simulink model "Lab_2v0"  (R2022a)
settings: Solver=VariableStepAuto  StartTime=0.0  StopTime=3600  RelTol=1e-12
settings Model: Creator=yjyoo  LastModifiedBy=ACL2022_14

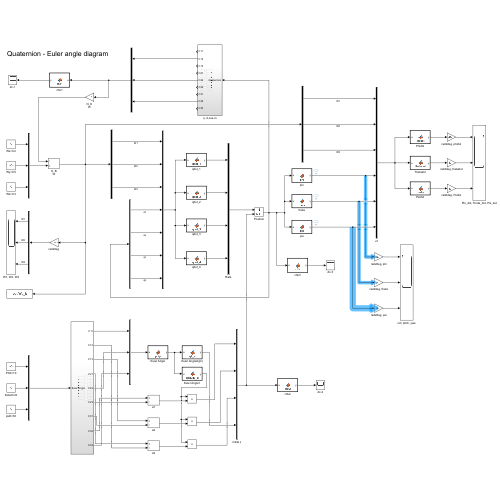
[thumbnail: Simulink's stored preview of the top-level diagram]
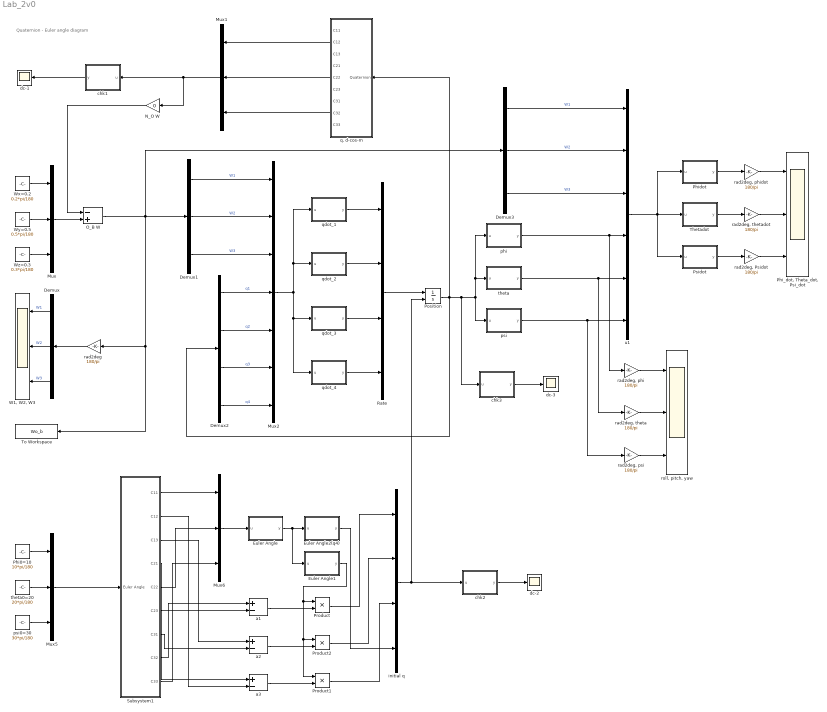
== system Lab_2v0 ==
  note: Quaternion - Euler angle diagram
  Demux : Demux  Outputs=3
  Demux1 : Demux  Outputs=3
  Demux2 : Demux
  Demux3 : Demux  Outputs=3
  Euler Angle : MATLAB Function  TreatAsAtomicUnit=on
  Euler Angle1 : MATLAB Function  TreatAsAtomicUnit=on
  Euler Angle2(q4) : MATLAB Function  TreatAsAtomicUnit=on
  Mux{,1,5..6} (4 alike) : Mux  Inputs=3
  Mux2 : Mux  Inputs=7
  N_O W : Gain  Gain=0
  O_B W : Sum  Inputs=-+
  Phi0=10 : Constant  Value=10*pi/180
  "Phi_dot, Theta_dot, Psi_dot" : Scope  NumInputPorts=3
  Phidot : MATLAB Function  TreatAsAtomicUnit=on
  Position : Integrator  InitialConditionSource=external
  Product : Product
  Product1 : Product
  Product2 : Product
  Psidot : MATLAB Function  TreatAsAtomicUnit=on
  Rate : Mux
  Subsystem1 : Subsystem
  Thetadot : MATLAB Function  TreatAsAtomicUnit=on
  To Workspace : ToWorkspace  VariableName=Wo_b  SaveFormat=Timeseries  SampleTime=-1
  "W1, W2, W3" : Scope  NumInputPorts=3
  Wx=0.2 : Constant  Value=0.2*pi/180
  Wy=0.5 : Constant  Value=0.5*pi/180
  Wz=0.3 : Constant  Value=0.3*pi/180
  a1 : Sum  Inputs=+-
  a2 : Sum  Inputs=+-
  a3 : Sum  Inputs=+-
  chk1 : MATLAB Function  TreatAsAtomicUnit=on
  chk2 : MATLAB Function  TreatAsAtomicUnit=on
  chk3 : MATLAB Function  TreatAsAtomicUnit=on
  dc-1 : Scope
  dc-2 : Scope
  dc-3 : Scope
  initial q : Mux
  phi : MATLAB Function  TreatAsAtomicUnit=on
  psi : MATLAB Function  TreatAsAtomicUnit=on
  psi0=30 : Constant  Value=30*pi/180
  q. d-cos-m : Subsystem
  qdot_1 : MATLAB Function  TreatAsAtomicUnit=on
  qdot_2 : MATLAB Function  TreatAsAtomicUnit=on
  qdot_3 : MATLAB Function  TreatAsAtomicUnit=on
  qdot_4 : MATLAB Function  TreatAsAtomicUnit=on
  rad2deg : Gain  Gain=180/pi
  "rad2deg, Psidot" : Gain  Gain=180/pi
  "rad2deg, phi" : Gain  Gain=180/pi
  "rad2deg, phidot" : Gain  Gain=180/pi
  "rad2deg, psi" : Gain  Gain=180/pi
  "rad2deg, theta" : Gain  Gain=180/pi
  "rad2deg, thetadot" : Gain  Gain=180/pi
  "roll, pitch, yaw" : Scope  NumInputPorts=3
  theta : MATLAB Function  TreatAsAtomicUnit=on
  theta0=20 : Constant  Value=20*pi/180
  u1 : Mux  Inputs=6
  wires:
  Wx=0.2/1 -> Mux/1
  Wy=0.5/1 -> Mux/2
  Wz=0.3/1 -> Mux/3
  Mux/1 -> O_B W/2
  N_O W/1 -> O_B W/1
  Mux1/1 -> N_O W/1, chk1/1(u)
  chk1/1(y) -> dc-1/1
  Demux/1 -> "W1, W2, W3"/1  "W1"
  Demux/2 -> "W1, W2, W3"/2  "W2"
  Demux/3 -> "W1, W2, W3"/3  "W3"
  O_B W/1 -> Demux1/1, Demux3/1, To Workspace/1, rad2deg/1
  Demux2/1 -> Mux2/4  "q1"
  Demux2/2 -> Mux2/5  "q2"
  Demux2/3 -> Mux2/6  "q3"
  Demux2/4 -> Mux2/7  "q4"
  Demux1/1 -> Mux2/1  "W1"
  Demux1/2 -> Mux2/2  "W2"
  Demux1/3 -> Mux2/3  "W3"
  rad2deg/1 -> Demux/1
  qdot_2/1(y) -> Rate/2
  qdot_1/1(y) -> Rate/1
  qdot_3/1(y) -> Rate/3
  qdot_4/1(y) -> Rate/4
  phi/1(y) -> "rad2deg, phi"/1, u1/4
  psi/1(y) -> "rad2deg, psi"/1, u1/6
  Demux3/1 -> u1/1  "W1"
  Demux3/2 -> u1/2  "W2"
  Demux3/3 -> u1/3  "W3"
  u1/1 -> Phidot/1(u), Psidot/1(u), Thetadot/1(u)
  "rad2deg, phidot"/1 -> "Phi_dot, Theta_dot, Psi_dot"/1
  "rad2deg, thetadot"/1 -> "Phi_dot, Theta_dot, Psi_dot"/2
  "rad2deg, Psidot"/1 -> "Phi_dot, Theta_dot, Psi_dot"/3
  Phidot/1(y) -> "rad2deg, phidot"/1
  Thetadot/1(y) -> "rad2deg, thetadot"/1
  Psidot/1(y) -> "rad2deg, Psidot"/1
  "rad2deg, psi"/1 -> "roll, pitch, yaw"/3
  "rad2deg, theta"/1 -> "roll, pitch, yaw"/2
  "rad2deg, phi"/1 -> "roll, pitch, yaw"/1
  theta/1(y) -> "rad2deg, theta"/1, u1/5
  Rate/1 -> Position/1
  Mux2/1 -> qdot_4/1(u), qdot_3/1(u), qdot_1/1(u), qdot_2/1(u)
  Position/1 -> Demux2/1, psi/1(u), phi/1(u), theta/1(u), chk3/1(u), q. d-cos-m/1(Quaternion)
  chk3/1(y) -> dc-3/1
  q. d-cos-m/2(C12) -> Mux1/1
  q. d-cos-m/5(C22) -> Mux1/2
  q. d-cos-m/8(C32) -> Mux1/3
  psi0=30/1 -> Mux5/3
  theta0=20/1 -> Mux5/2
  Phi0=10/1 -> Mux5/1
  Mux5/1 -> Subsystem1/1(Euler Angle)
  Mux6/1 -> Euler Angle/1(u)
  initial q/1 -> Position/2, chk2/1(u)
  chk2/1(y) -> dc-2/1
  Euler Angle2(q4)/1(y) -> initial q/4
  Euler Angle1/1(y) -> Product2/1, Product1/1, Product/1
  a1/1 -> Product/2
  a2/1 -> Product2/2
  a3/1 -> Product1/2
  Product/1 -> initial q/1
  Product2/1 -> initial q/2
  Product1/1 -> initial q/3
  Euler Angle/1(y) -> Euler Angle1/1(u), Euler Angle2(q4)/1(u)
  Subsystem1/8(C32) -> a1/1
  Subsystem1/6(C23) -> a1/2
  Subsystem1/3(C13) -> a2/1
  Subsystem1/7(C31) -> a2/2
  Subsystem1/4(C21) -> a3/1
  Subsystem1/2(C12) -> a3/2
  Subsystem1/1(C11) -> Mux6/1
  Subsystem1/5(C22) -> Mux6/2
  Subsystem1/9(C33) -> Mux6/3

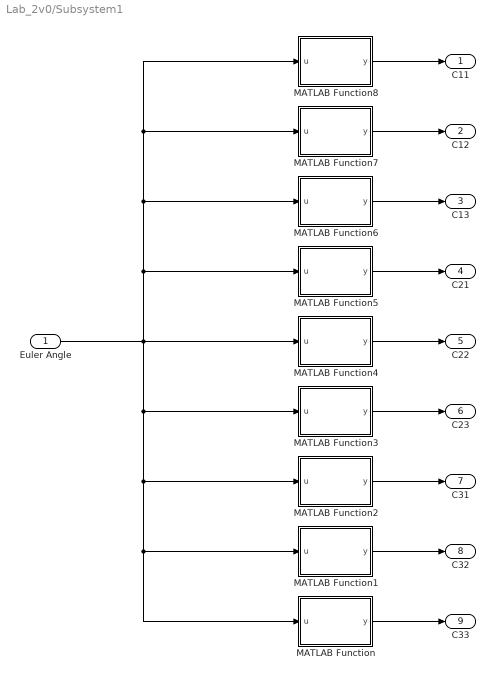
== system Lab_2v0/Subsystem1 ==
  Euler Angle : Inport
  MATLAB Function : MATLAB Function  TreatAsAtomicUnit=on
  MATLAB Function1 : MATLAB Function  TreatAsAtomicUnit=on
  MATLAB Function2 : MATLAB Function  TreatAsAtomicUnit=on
  MATLAB Function3 : MATLAB Function  TreatAsAtomicUnit=on
  MATLAB Function4 : MATLAB Function  TreatAsAtomicUnit=on
  MATLAB Function5 : MATLAB Function  TreatAsAtomicUnit=on
  MATLAB Function6 : MATLAB Function  TreatAsAtomicUnit=on
  MATLAB Function7 : MATLAB Function  TreatAsAtomicUnit=on
  MATLAB Function8 : MATLAB Function  TreatAsAtomicUnit=on
  C11 : Outport
  C12 : Outport  Port=2
  C13 : Outport  Port=3
  C21 : Outport  Port=4
  C22 : Outport  Port=5
  C23 : Outport  Port=6
  C31 : Outport  Port=7
  C32 : Outport  Port=8
  C33 : Outport  Port=9
  wires:
  Euler Angle/1 -> MATLAB Function/1(u), MATLAB Function1/1(u), MATLAB Function2/1(u), MATLAB Function3/1(u), MATLAB Function8/1(u), MATLAB Function7/1(u), MATLAB Function6/1(u), MATLAB Function5/1(u), MATLAB Function4/1(u)
  MATLAB Function/1(y) -> C33/1
  MATLAB Function1/1(y) -> C32/1
  MATLAB Function2/1(y) -> C31/1
  MATLAB Function3/1(y) -> C23/1
  MATLAB Function4/1(y) -> C22/1
  MATLAB Function5/1(y) -> C21/1
  MATLAB Function6/1(y) -> C13/1
  MATLAB Function7/1(y) -> C12/1
  MATLAB Function8/1(y) -> C11/1

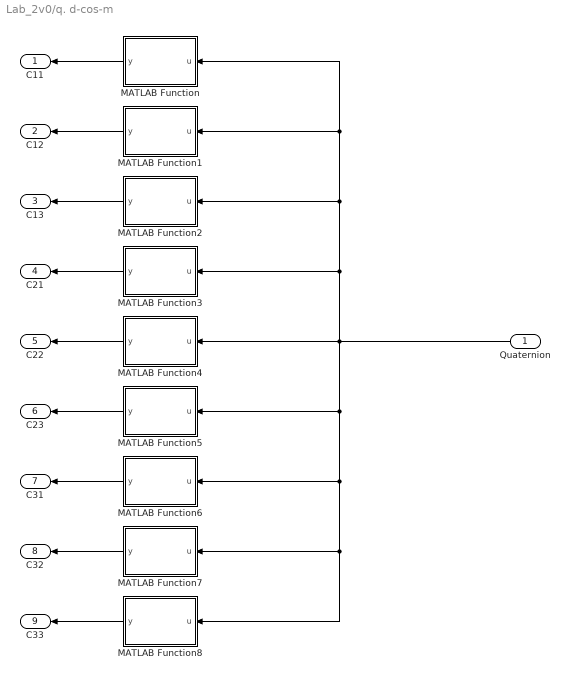
== system Lab_2v0/q. d-cos-m ==
  Quaternion : Inport
  MATLAB Function : MATLAB Function  TreatAsAtomicUnit=on
  MATLAB Function1 : MATLAB Function  TreatAsAtomicUnit=on
  MATLAB Function2 : MATLAB Function  TreatAsAtomicUnit=on
  MATLAB Function3 : MATLAB Function  TreatAsAtomicUnit=on
  MATLAB Function4 : MATLAB Function  TreatAsAtomicUnit=on
  MATLAB Function5 : MATLAB Function  TreatAsAtomicUnit=on
  MATLAB Function6 : MATLAB Function  TreatAsAtomicUnit=on
  MATLAB Function7 : MATLAB Function  TreatAsAtomicUnit=on
  MATLAB Function8 : MATLAB Function  TreatAsAtomicUnit=on
  C11 : Outport
  C12 : Outport  Port=2
  C13 : Outport  Port=3
  C21 : Outport  Port=4
  C22 : Outport  Port=5
  C23 : Outport  Port=6
  C31 : Outport  Port=7
  C32 : Outport  Port=8
  C33 : Outport  Port=9
  wires:
  Quaternion/1 -> MATLAB Function8/1(u), MATLAB Function7/1(u), MATLAB Function6/1(u), MATLAB Function5/1(u), MATLAB Function3/1(u), MATLAB Function/1(u), MATLAB Function1/1(u), MATLAB Function2/1(u), MATLAB Function4/1(u)
  MATLAB Function/1(y) -> C11/1
  MATLAB Function1/1(y) -> C12/1
  MATLAB Function2/1(y) -> C13/1
  MATLAB Function3/1(y) -> C21/1
  MATLAB Function4/1(y) -> C22/1
  MATLAB Function5/1(y) -> C23/1
  MATLAB Function6/1(y) -> C31/1
  MATLAB Function7/1(y) -> C32/1
  MATLAB Function8/1(y) -> C33/1

== matlab function Lab_2v0/qdot_1 ==
  data: u input; y output
function y = qdot_1(u)

y = 0.5*(u(3)*u(5) - u(2)*u(6) + u(1)*u(7));

end

== matlab function Lab_2v0/q. d-cos-m/MATLAB Function1 ==
  data: u input; y output
function y = C12(u)

y = 2*(u(1)*u(2) + u(3)*u(4));

end

== matlab function Lab_2v0/q. d-cos-m/MATLAB Function2 ==
  data: u input; y output
function y = C13(u)

y = 2*(u(1)*u(3) - u(2)*u(4));

end

== matlab function Lab_2v0/q. d-cos-m/MATLAB Function3 ==
  data: u input; y output
function y = C21(u)

y = 2*(u(1)*u(2) - u(3)*u(4));

end

== matlab function Lab_2v0/q. d-cos-m/MATLAB Function4 ==
  data: u input; y output
function y = C22(u)

y = -u(1)^2 + u(2)^2 - u(3)^2 + u(4)^2;

end

== matlab function Lab_2v0/q. d-cos-m/MATLAB Function5 ==
  data: u input; y output
function y = C23(u)

y = 2*(u(2)*u(3) + u(1)*u(4));

end

== matlab function Lab_2v0/q. d-cos-m/MATLAB Function6 ==
  data: u input; y output
function y = C31(u)

y = 2*(u(1)*u(3) + u(2)*u(4));

end

== matlab function Lab_2v0/q. d-cos-m/MATLAB Function7 ==
  data: u input; y output
function y = C32(u)

y = 2*(u(2)*u(3) - u(1)*u(4));

end

== matlab function Lab_2v0/q. d-cos-m/MATLAB Function8 ==
  data: u input; y output
function y = C33(u)

y = -u(1)^2 - u(2)^2 + u(3)^2 +u(4)^2;

end

== matlab function Lab_2v0/Subsystem1/MATLAB Function ==
  data: u input; y output
function y = c33_e(u)

y = cos(u(2))*cos(u(1));

end

== matlab function Lab_2v0/Subsystem1/MATLAB Function1 ==
  data: u input; y output
function y = c32_e(u)

y = -cos(u(3))*sin(u(1)) + sin(u(3))*sin(u(2))*cos(u(1));

end

== matlab function Lab_2v0/chk1 ==
  data: u input; y output
function y = chk1(u)

y = u(1)^2 + u(2)^2 + u(3)^2;

end

== matlab function Lab_2v0/Subsystem1/MATLAB Function2 ==
  data: u input; y output
function y = c31_e(u)

y = sin(u(3))*sin(u(1)) + cos(u(3))*sin(u(2))*cos(u(1));

end

== matlab function Lab_2v0/Subsystem1/MATLAB Function3 ==
  data: u input; y output
function y = c23_e(u)

y = cos(u(2))*sin(u(1));

end

== matlab function Lab_2v0/Subsystem1/MATLAB Function4 ==
  data: u input; y output
function y = c22_e(u)

y = cos(u(3))*cos(u(1)) + sin(u(3))*sin(u(2))*sin(u(1));

end

== matlab function Lab_2v0/Subsystem1/MATLAB Function5 ==
  data: u input; y output
function y = c21_e(u)

y = -sin(u(3))*cos(u(1)) + cos(u(3))*sin(u(2))*sin(u(1));

end

== matlab function Lab_2v0/Subsystem1/MATLAB Function6 ==
  data: u input; y output
function y = c13_e(u)

y = -sin(u(2));

end

== matlab function Lab_2v0/Subsystem1/MATLAB Function7 ==
  data: u input; y output
function y = c12_e(u)

y = sin(u(3))*cos(u(2));

end

== matlab function Lab_2v0/Subsystem1/MATLAB Function8 ==
  data: u input; y output
function y = c11_e(u)

y = cos(u(3))*cos(u(2));

end

== matlab function Lab_2v0/Euler Angle ==
  data: u input; y output
function y = phip(u)

y = acos((u(1)+u(2)+u(3)-1)/2);

end

== matlab function Lab_2v0/Euler Angle1 ==
  data: u input; y output
function y = q1q2q3_e(u)

y = 1/(4*cos(u/2));

end

== matlab function Lab_2v0/Euler Angle2(q4) ==
  data: u input; y output
function y = q4_e(u)

y = cos(u/2);

end

== matlab function Lab_2v0/qdot_2 ==
  data: u input; y output


function y = qdot_2(u)

y = 0.5*(-u(3)*u(4)+u(1)*u(6)+u(2)*u(7));

end

== matlab function Lab_2v0/chk2 ==
  data: u input; y output
function y = chk2(u)

y = u(1)^2 + u(2)^2 + u(3)^2 + u(4)^2;

end

== matlab function Lab_2v0/qdot_3 ==
  data: u input; y output
function y = qdot_3(u)

y = 0.5*(u(2)*u(4) -u(1)*u(5) + u(3)*u(7));

end

== matlab function Lab_2v0/qdot_4 ==
  data: u input; y output
function y = qdot_4(u)

y = 0.5*(-u(1)*u(4) - u(2)*u(5) - u(3)*u(6));

end

== matlab function Lab_2v0/chk3 ==
  data: u input; y output
function y = chk(u)

y = u(1)^2 + u(2)^2 + u(3)^2 + u(4)^2;

end

== matlab function Lab_2v0/phi ==
  data: u input; y output
function y = phi(u)

y = atan((2*u(1)*u(4) + u(2)*u(3))/(1-2*(u(1)^2 + u(2)^2)));

end

== matlab function Lab_2v0/theta ==
  data: u input; y output
function y = theta(u)

y = asin(2*(u(2)*u(4) - u(3)*u(1)));

end

== matlab function Lab_2v0/psi ==
  data: u input; y output
function y = psi(u)

y = atan((2*(u(3)*u(4) + u(1)*u(2)))/(1-2*(u(2)^2+u(3)^2)));

end

== matlab function Lab_2v0/Thetadot ==
  data: u input; y output
function y = thetadot(u)

y = cos(u(4))*u(2) - sin(u(4))*u(3);

end

== matlab function Lab_2v0/Psidot ==
  data: u input; y output
function y = psidot(u)

y = (sin(u(4))/cos(u(5)))*u(2) + (cos(u(4))/cos(u(5)))*u(3);

end

== matlab function Lab_2v0/Phidot ==
  data: u input; y output
function y = phidot(u)

y = u(1) + sin(u(4))*tan(u(5))*u(2) + cos(u(4))*tan(u(5))*u(3);

end

== matlab function Lab_2v0/q. d-cos-m/MATLAB Function ==
  data: u input; y output
function y = C11(u)

y = u(1)^2 - u(2)^2 - u(3)^2 + u(4)^2;

end
